simulink library "asbhl20airdata"  (R2016b)
settings: Solver=VariableStepAuto  StartTime=0.0  StopTime=10.0  RelTol=1e-3
undefined symbols (not defined in the file): Tc, Ts
Description:
  | HL-20 air data computer signal marshaling component module
  | 
  | Copyright 1990-2005 The MathWorks Inc.
settings Model: Creator=The MathWorks, Inc.  LastModifiedBy=The MathWorks, Inc.
settings DataIOCC: SaveFormat=Array  SignalLoggingSaveFormat=ModelDataLogs
settings OptimizationCC: BlockReduction=off  BooleanDataType=off
settings DebuggingCC: SaveWithParameterizedLinksMsg=none  UnderspecifiedInitializationDetection=Classic  MergeDetectMultiDrivingBlocksExec=none  SignalResolutionControl=TryResolveAllWithWarning  MultiTaskCondExecSysMsg=none  StrictBusMsg=None
settings HardwareCC: ProdBitPerPointer=32  ProdBitPerSizeT=32  ProdBitPerPtrDiffT=32  ProdLargestAtomicFloat=None  ProdIntDivRoundTo=Undefined  ProdEndianess=Unspecified  ProdWordSize=32  ProdHWDeviceType=32-bit Generic  TargetUnknown=on
settings ModelReferenceCC: PropagateSignalLabelsOutOfModel=off
settings ConfigComp: CovMetricSettings=dw  CovHtmlReporting=on  CovSaveCumulativeToWorkspaceVar=on  CovSaveSingleToWorkspaceVar=on  CovExternalEMLEnable=off

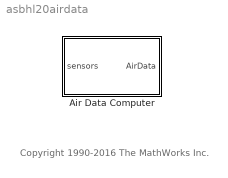
== system asbhl20airdata ==
  note: Copyright 1990-2016 The MathWorks Inc.
  Air Data Computer : Subsystem  TreatAsAtomicUnit=on

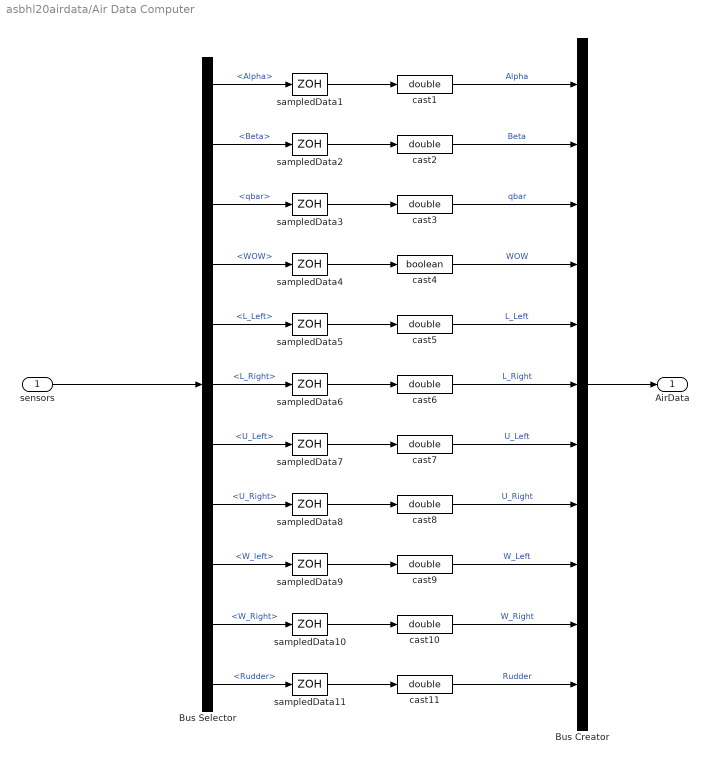
== system asbhl20airdata/Air Data Computer ==
  sensors : Inport  SampleTime=Ts
  Bus Creator : BusCreator  Inputs=11  OutDataTypeStr=Bus: AirDataBus
  Bus Selector : BusSelector  OutputSignals=Alpha,Beta,qbar,LGData.WOW,Act_positions.L_Left,Act_positions.L_Right,Act_positions.U_Left,Act_positions.U_Right,Act_positions.W_left,Act_positions.W_Right,Act_positions.Rudder
  cast{1..3,5..11} (10 alike) : DataTypeConversion  OutDataTypeStr=double
  cast4 : DataTypeConversion  OutDataTypeStr=boolean
  sampledData{1..11} (11 alike) : ZeroOrderHold  SampleTime=Tc
  AirData : Outport
  wires:
  sensors/1 -> Bus Selector/1
  Bus Selector/1 -> sampledData1/1  "<Alpha>"
  Bus Selector/2 -> sampledData2/1  "<Beta>"
  Bus Creator/1 -> AirData/1
  cast1/1 -> Bus Creator/1  "Alpha"
  cast2/1 -> Bus Creator/2  "Beta"
  Bus Selector/3 -> sampledData3/1  "<qbar>"
  cast3/1 -> Bus Creator/3  "qbar"
  Bus Selector/4 -> sampledData4/1  "<WOW>"
  cast11/1 -> Bus Creator/11  "Rudder"
  cast10/1 -> Bus Creator/10  "W_Right"
  cast9/1 -> Bus Creator/9  "W_Left"
  Bus Selector/11 -> sampledData11/1  "<Rudder>"
  Bus Selector/10 -> sampledData10/1  "<W_Right>"
  Bus Selector/9 -> sampledData9/1  "<W_left>"
  Bus Selector/8 -> sampledData8/1  "<U_Right>"
  cast8/1 -> Bus Creator/8  "U_Right"
  Bus Selector/7 -> sampledData7/1  "<U_Left>"
  cast7/1 -> Bus Creator/7  "U_Left"
  cast6/1 -> Bus Creator/6  "L_Right"
  Bus Selector/6 -> sampledData6/1  "<L_Right>"
  cast5/1 -> Bus Creator/5  "L_Left"
  Bus Selector/5 -> sampledData5/1  "<L_Left>"
  sampledData1/1 -> cast1/1
  sampledData2/1 -> cast2/1
  sampledData3/1 -> cast3/1
  sampledData4/1 -> cast4/1
  sampledData5/1 -> cast5/1
  sampledData6/1 -> cast6/1
  sampledData7/1 -> cast7/1
  sampledData8/1 -> cast8/1
  sampledData9/1 -> cast9/1
  sampledData10/1 -> cast10/1
  sampledData11/1 -> cast11/1
  cast4/1 -> Bus Creator/4  "WOW"
